simulink model "rolling_motion"  (R2017b)
settings: Solver=VariableStepAuto  StartTime=0.0  StopTime=runtime  RelTol=1e-3
values from neighbouring files (symbols this model uses):
  Kp = 10    [rolling_motion_runscript.m]
  Lda = 20    [EKF_Param_Est.m]    (also in KF_Generic_Test.m = L(2); KFex2D.m = 116; SysID.m = L(2); gncEx_LS.m = L(2))
  Lp = -10    [EKF_Param_Est.m]    (also in KF_Generic_Test.m = L(1); KFex2D.m = -9; SysID.m = L(1); gncEx_LS.m = L(1))
  Td = 0    [rolling_motion_runscript.m]
  Ti = 1000000    [rolling_motion_runscript.m]
  uamp = 1    [rolling_motion_runscript.m]
  ufreq = 1    [rolling_motion_runscript.m]
libraries: simulink x1
settings Model: Creator=stroll  LastModifiedBy=stroll

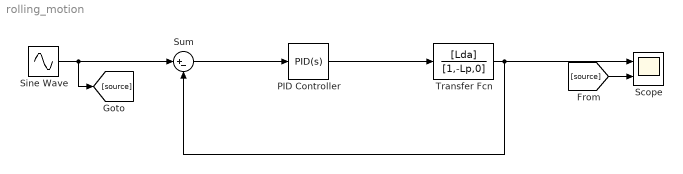
== system rolling_motion ==
  PID Controller : simulink/Continuous/PID Controller  Controller=PID  TimeDomain=Continuous-time  SampleTime=-1  IntegratorMethod=Forward Euler  FilterMethod=Forward Euler  Form=Parallel  UseFilter=on  ControllerParametersSource=internal  P=Kp  I=Kp/Ti  D=Kp*Td  N=100  InitialConditionSource=internal  InitialConditionForIntegrator=0  InitialConditionForFilter=0  ExternalReset=none  LimitOutput=off  UpperSaturationLimit=inf  LowerSaturationLimit=-inf  LinearizeAsGain=on  AntiWindupMode=none  Kb=1  TrackingMode=off  Kt=1  PParamMin=[]  PParamMax=[]  IParamMin=[]  IParamMax=[]  DParamMin=[]  DParamMax=[]  NParamMin=[]  NParamMax=[]  KbParamMin=[]  KbParamMax=[]  KtParamMin=[]  KtParamMax=[]  POutMin=[]  POutMax=[]  IOutMin=[]  IOutMax=[]  DOutMin=[]  DOutMax=[]  NOutMin=[]  NOutMax=[]  KbOutMin=[]  KbOutMax=[]  KtOutMin=[]  KtOutMax=[]  IntegratorOutMin=[]  IntegratorOutMax=[]  FilterOutMin=[]  FilterOutMax=[]  SumOutMin=[]  SumOutMax=[]  SumI1OutMin=[]  SumI1OutMax=[]  SumI2OutMin=[]  SumI2OutMax=[]  SumI3OutMin=[]  SumI3OutMax=[]  SumDOutMin=[]  SumDOutMax=[]  SaturationOutMin=[]  SaturationOutMax=[]  IntegratorContinuousStateAttributes=''  IntegratorStateMustResolveToSignalObject=off  IntegratorRTWStateStorageClass=Auto  FilterContinuousStateAttributes=''  FilterStateMustResolveToSignalObject=off  FilterRTWStateStorageClass=Auto  DifferentiatorICPrevScaledInput=0  DifferentiatorOutMin=[]  DifferentiatorOutMax=[]  InitialConditionSetting=State (most efficient)  FilterDiffOutCoefMin=[]  FilterDiffOutCoefMax=[]  SumDenOutMin=[]  SumDenOutMax=[]  SumNumOutMin=[]  SumNumOutMax=[]  ReciprocalOutMin=[]  ReciprocalOutMax=[]  DivideOutMin=[]  DivideOutMax=[]  TunerSelectOption=Transfer Function Based (PID Tuner App)
  Scope : Scope  NumInputPorts=2
  Sine Wave : Sin  Amplitude=uamp  Frequency=ufreq  SampleTime=0
  Sum : Sum  Inputs=|+-
  Transfer Fcn : TransferFcn  Numerator=[Lda]  Denominator=[1,-Lp,0]
  wires:
  Transfer Fcn/1 -> Sum/2, Scope/1
  [source] -> Scope/2
  Sum/1 -> PID Controller/1
  PID Controller/1 -> Transfer Fcn/1
  Sine Wave/1 -> [source], Sum/1
